simulink model "JointSpaceGravityCompensation"  (R2022b)
settings: Solver=VariableStepAuto  StartTime=0.0  StopTime=10.0  RelTol=1e-3
values from neighbouring files (symbols this model uses):
  Fc = 1    [parameters.m]
  Kd = [[10,0,0] ... (first row only)    [parameters.m]
  Kp = [[100,0,0] ... (first row only)    [parameters.m]
  qd = [1.3, -0.25, -1.3]    [parameters.m]
settings Model: Creator=uzair  LastModifiedBy=uzair

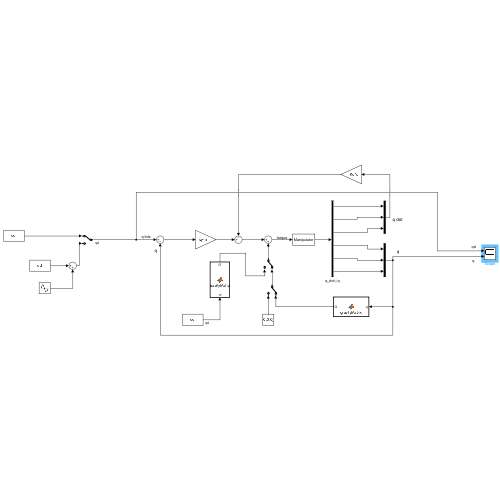
[thumbnail: Simulink's stored preview of the top-level diagram]
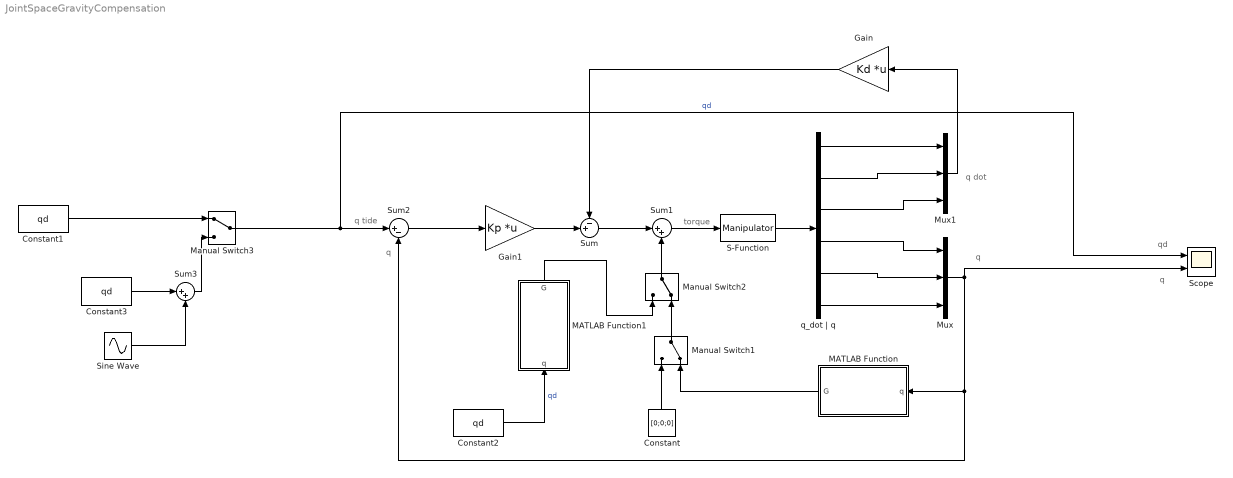
== system JointSpaceGravityCompensation ==
  note: torque
  note: q tide
  note: q
  note: qd
  note: q
  note: q dot
  note: q
  Constant : Constant  Value=[0;0;0]
  Constant1 : Constant  Value=qd
  Constant2 : Constant  Value=qd
  Constant3 : Constant  Value=qd
  Gain : Gain  Gain=Kd  Multiplication=Matrix(K*u)
  Gain1 : Gain  Gain=Kp  Multiplication=Matrix(K*u)
  MATLAB Function : MATLAB Function  TreatAsAtomicUnit=on
  MATLAB Function1 : MATLAB Function  TreatAsAtomicUnit=on
  Manual Switch1 : ManualSwitch  CurrentSetting=0
  Manual Switch2 : ManualSwitch  CurrentSetting=0
  Manual Switch3 : ManualSwitch
  Mux : Mux  Inputs=3
  Mux1 : Mux  Inputs=3
  S-Function : S-Function  FunctionName=Manipulator  Parameters=params  SFunctionDeploymentMode=off  EnableBusSupport=off
  Scope : Scope  NumInputPorts=2
  Sine Wave : Sin  Amplitude=0.5  Frequency=2*pi*Fc  SampleTime=0
  Sum : Sum  Inputs=-+|
  Sum1 : Sum  Inputs=|++
  Sum2 : Sum  Inputs=|+-
  Sum3 : Sum  Inputs=|++
  q_dot | q : Demux  Outputs=6
  wires:
  S-Function/1 -> q_dot | q/1
  q_dot | q/6 -> Mux/3
  q_dot | q/5 -> Mux/2
  q_dot | q/4 -> Mux/1
  q_dot | q/1 -> Mux1/1
  q_dot | q/2 -> Mux1/2
  q_dot | q/3 -> Mux1/3
  Mux1/1 -> Gain/1
  Gain/1 -> Sum/1
  Sum/1 -> Sum1/1
  Sum1/1 -> S-Function/1
  Mux/1 -> Scope/2, Sum2/2, MATLAB Function/1(q)
  Gain1/1 -> Sum/2
  Sum2/1 -> Gain1/1
  Manual Switch3/1 -> Scope/1, Sum2/1  "qd"
  MATLAB Function/1(G) -> Manual Switch1/2
  Constant/1 -> Manual Switch1/1
  Manual Switch1/1 -> Manual Switch2/2
  MATLAB Function1/1(G) -> Manual Switch2/1
  Constant2/1 -> MATLAB Function1/1(q)  "qd"
  Manual Switch2/1 -> Sum1/2
  Sine Wave/1 -> Sum3/2
  Constant3/1 -> Sum3/1
  Sum3/1 -> Manual Switch3/2
  Constant1/1 -> Manual Switch3/1

== matlab function JointSpaceGravityCompensation/MATLAB Function ==
  data: q input; G output
function G = gravityMatrix(q)
    q1 = q(1);
    q2 = q(2);
    q3 = q(3);
    G = [(1720953*cos(q1))/781250 - (6751431*sin(q1))/6250000 + (264762*cos(q1)*cos(q3))/1953125 + (132381*pi*cos(q1))/156250 - (1720953*q2*sin(q1))/312500;
                                                                                                                          (1720953*cos(q1))/312500;
                                                                                                                 -(264762*sin(q1)*sin(q3))/1953125];
end

== matlab function JointSpaceGravityCompensation/MATLAB Function1 ==
  data: q input; G output
function G = gravityMatrix(q)
    q1 = q(1);
    q2 = q(2);
    q3 = q(3);
    G = [(1720953*cos(q1))/781250 - (6751431*sin(q1))/6250000 + (264762*cos(q1)*cos(q3))/1953125 + (132381*pi*cos(q1))/156250 - (1720953*q2*sin(q1))/312500;
                                                                                                                          (1720953*cos(q1))/312500;
                                                                                                                 -(264762*sin(q1)*sin(q3))/1953125];
end
